simulink model "DesigningofBuckBoostChopper"  (Simulink 7.3)
settings: Solver=ode45  StartTime=0.0  StopTime=0.1  RelTol=1e-3
libraries: powerlib x9, powerlib_extras x1
settings Model: Creator=srija  LastModifiedBy=srija

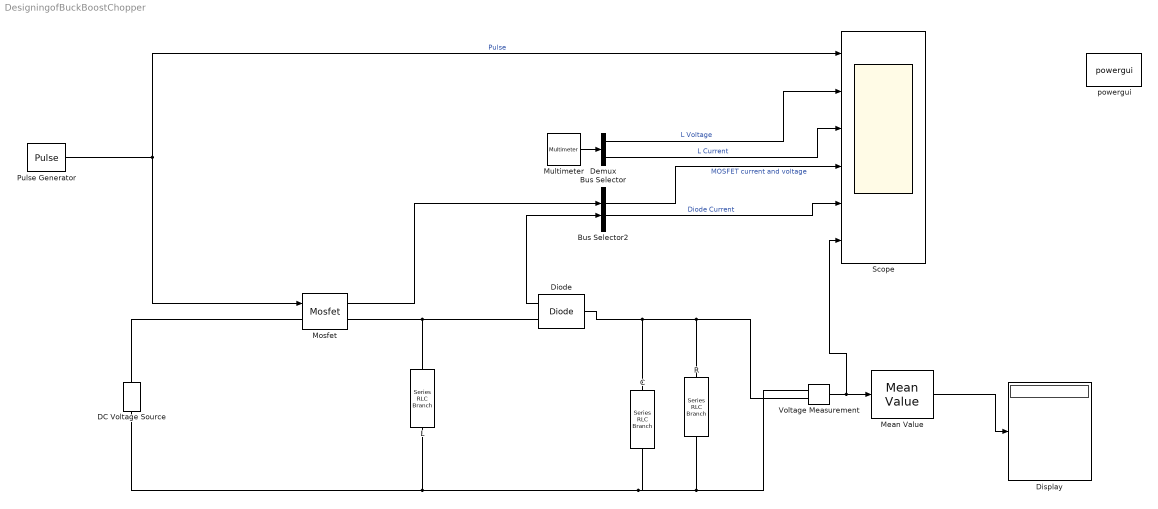
== system DesigningofBuckBoostChopper ==
  Bus Selector : BusSelector  OutputSignals=MOSFET current,MOSFET voltage  OutputAsBus=on
  Bus Selector2 : BusSelector  OutputSignals=Diode current  OutputAsBus=on
  C : powerlib/Elements/Series RLC Branch  DialogController=POWERSYS.PowerSysDialog  PhysicalDomain=powersysdomain  SubClassName=unknown  LeftPortType=p1  RightPortType=p1  LConnTagsString=__new0  RConnTagsString=__new0  BranchType=C  Resistance=1  Inductance=1e-3  SetiL0=off  InitialCurrent=0  Capacitance=833e-6  Setx0=off  InitialVoltage=0  Measurements=None
  DC Voltage Source : powerlib/Electrical Sources/DC Voltage Source  DialogController=POWERSYS.PowerSysDialog  SystemSampleTime=-1  Amplitude=20  Measurements=None
  Demux : Demux  Outputs=2
  Diode : powerlib/Power Electronics/Diode  DialogController=POWERSYS.PowerSysDialog  SystemSampleTime=-1  Ron=0.000001  Lon=0  Vf=0  IC=0  UseSnubber=off  Rs=500  Cs=250e-9  Measurements=on
  Display : Display
  L : powerlib/Elements/Series RLC Branch  DialogController=POWERSYS.PowerSysDialog  PhysicalDomain=powersysdomain  SubClassName=unknown  LeftPortType=p1  RightPortType=p1  LConnTagsString=__new0  RConnTagsString=__new0  BranchType=L  Resistance=1  Inductance=111e-6  SetiL0=off  InitialCurrent=0  Capacitance=1e-6  Setx0=off  InitialVoltage=0  Measurements=Branch voltage and current
  Mean Value : powerlib_extras/Measurements/Mean Value  DialogController=POWERSYS.PowerSysDialog  SystemSampleTime=-1  Period=50e-6
  Mosfet : powerlib/Power Electronics/Mosfet  DialogController=POWERSYS.PowerSysDialog  SystemSampleTime=-1  Ron=0.00000001  Lon=0  Rd=0.0000001  Vfd=0  IC=0  Rs=1e5  Cs=inf  Measurements=on
  Multimeter : powerlib/Measurements/Multimeter  SystemSampleTime=-1  PhasorSimulation=off  OutputType=Complex  sel=[1 2]  L=2  Gain=[1 1]  yselected={'Ub: L','Ib: L'};  PSBOutputType=1  PSBequivalent=0  AxesSetting=[0,0.1,-100,100]  Display=0  SavedBlockNames=-11
  Pulse Generator : DiscretePulseGenerator  PulseType=Time based  Amplitude=1  Period=50e-6  PulseWidth=66  PhaseDelay=0  SampleTime=1
  R : powerlib/Elements/Series RLC Branch  DialogController=POWERSYS.PowerSysDialog  PhysicalDomain=powersysdomain  SubClassName=unknown  LeftPortType=p1  RightPortType=p1  LConnTagsString=__new0  RConnTagsString=__new0  BranchType=R  Resistance=10  Inductance=1e-3  SetiL0=off  InitialCurrent=0  Capacitance=1e-6  Setx0=off  InitialVoltage=0  Measurements=None
  Scope : Scope  NumInputPorts=6
      settings: TimeRange=0.02500000000000001  YMin=0~-20~-16~0~0~38.7  YMax=1~40~-8~60~15~39
  Voltage Measurement : powerlib/Measurements/Voltage Measurement  DialogController=POWERSYS.PowerSysDialog  SystemSampleTime=-1  PhasorSimulation=off  OutputType=Complex  PSBequivalent=0
  powergui : powerlib/powergui  Priority=1  SystemSampleTime=-1  SimulationMode=Continuous  SampleTime=50e-6  frequency=60  SPID=off  DisableSnubberDevices=off  DisableRonSwitches=off  DisableVfSwitches=off  SwTol=0  Interpol=off  frequencyindice=0  echomessages=off  HookPort=off  DisplayEquations=off  FunctionMessages=off  EnableUseOfTLC=off  x0status=blocks  RestoreLinks=warning  Frange=[0:2:500]  Ylog=off  Xlog=on  ShowGrid=off  save=off  variable=ZData  ZoomFFT=on  StartTime=0.0  cycles=1  DisplayStyle=1  fundamental=60  FreqAxis=off  MaxFrequency=1000  frequencyindicesteady=1  RmsSteady=1  display=off  Ts=0  methode=off
  wires:
  Voltage Measurement/1 -> Mean Value/1, Scope/6
  Mean Value/1 -> Display/1
  Multimeter/1 -> Demux/1
  Demux/1 -> Scope/2  "L Voltage"
  Demux/2 -> Scope/3  "L Current"
  Pulse Generator/1 -> Mosfet/1, Scope/1  "Pulse"
  Mosfet/1 -> Bus Selector/1
  Bus Selector/1 -> Scope/4  "MOSFET current and voltage"
  Diode/1 -> Bus Selector2/1
  Bus Selector2/1 -> Scope/5  "Diode Current"
  connections:
  DC Voltage Source/RConn1 -- Mosfet/LConn1
  L/RConn1 -- Mosfet/RConn1 -- Diode/RConn1
  R/RConn1 -- L/LConn1 -- DC Voltage Source/LConn1 -- C/RConn1 -- Voltage Measurement/LConn1
  C/LConn1 -- Diode/LConn1 -- R/LConn1 -- Voltage Measurement/LConn2
